simulink model "attitude_sysid"  (R2018a)
settings: Solver=VariableStepAuto  StartTime=0.0  StopTime=40  RelTol=1e-3
undefined symbols (not defined in the file): drone, simulation_sampling_ts
libraries: simulink x4
settings Model: Creator=ros  LastModifiedBy=ros

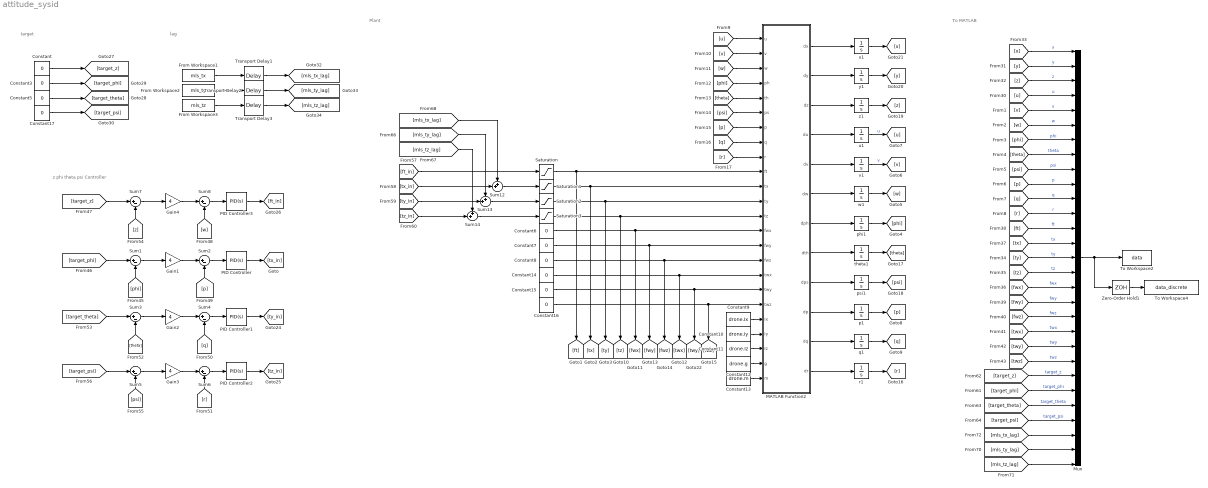
== system attitude_sysid ==
  note: Plant
  note: target
  note: lag
  note: z phi theta psi Controller
  note: To MATLAB
  Constant{,3,5..8,14..17} (10 alike) : Constant  Value=0
  Constant10 : Constant  Value=drone.Iy
  Constant11 : Constant  Value=drone.Iz
  Constant12 : Constant  Value=drone.g
  Constant13 : Constant  Value=drone.m
  Constant9 : Constant  Value=drone.Ix
  From Workspace1 : FromWorkspace  VariableName=mls_tx  SampleTime=0
  From Workspace2 : FromWorkspace  VariableName=mls_ty  SampleTime=0
  From Workspace3 : FromWorkspace  VariableName=mls_tz  SampleTime=0
  Gain{1..4} (4 alike) : Gain  Gain=4
  MATLAB Function2 : MATLAB Function  TreatAsAtomicUnit=on
  Mux : Mux  Inputs=29
  PID Controller : simulink/Continuous/PID Controller  Controller=PID  TimeDomain=Continuous-time  SampleTime=-1  IntegratorMethod=Forward Euler  FilterMethod=Forward Euler  Form=Parallel  UseFilter=on  ControllerParametersSource=internal  P=1.5  I=1.5  D=0  N=100  InitialConditionSource=internal  InitialConditionForIntegrator=0  InitialConditionForFilter=0  ExternalReset=none  LimitOutput=off  UpperSaturationLimit=inf  LowerSaturationLimit=-inf  LinearizeAsGain=on  AntiWindupMode=none  Kb=1  TrackingMode=off  Kt=1  PParamMin=[]  PParamMax=[]  IParamMin=[]  IParamMax=[]  DParamMin=[]  DParamMax=[]  NParamMin=[]  NParamMax=[]  KbParamMin=[]  KbParamMax=[]  KtParamMin=[]  KtParamMax=[]  POutMin=[]  POutMax=[]  IOutMin=[]  IOutMax=[]  DOutMin=[]  DOutMax=[]  NOutMin=[]  NOutMax=[]  KbOutMin=[]  KbOutMax=[]  KtOutMin=[]  KtOutMax=[]  IntegratorOutMin=[]  IntegratorOutMax=[]  FilterOutMin=[]  FilterOutMax=[]  SumOutMin=[]  SumOutMax=[]  SumI1OutMin=[]  SumI1OutMax=[]  SumI2OutMin=[]  SumI2OutMax=[]  SumI3OutMin=[]  SumI3OutMax=[]  SumDOutMin=[]  SumDOutMax=[]  SaturationOutMin=[]  SaturationOutMax=[]  IntegratorContinuousStateAttributes=''  IntegratorStateMustResolveToSignalObject=off  IntegratorRTWStateStorageClass=Auto  FilterContinuousStateAttributes=''  FilterStateMustResolveToSignalObject=off  FilterRTWStateStorageClass=Auto  DifferentiatorICPrevScaledInput=0  DifferentiatorOutMin=[]  DifferentiatorOutMax=[]  FilterDiffOutCoefMin=[]  FilterDiffOutCoefMax=[]  SumDenOutMin=[]  SumDenOutMax=[]  SumNumOutMin=[]  SumNumOutMax=[]  ReciprocalOutMin=[]  ReciprocalOutMax=[]  DivideOutMin=[]  DivideOutMax=[]  TunerSelectOption=Transfer Function Based (PID Tuner App)
  PID Controller1 : simulink/Continuous/PID Controller  Controller=PID  TimeDomain=Continuous-time  SampleTime=-1  IntegratorMethod=Forward Euler  FilterMethod=Forward Euler  Form=Parallel  UseFilter=on  ControllerParametersSource=internal  P=1.5  I=1.5  D=0  N=100  InitialConditionSource=internal  InitialConditionForIntegrator=0  InitialConditionForFilter=0  ExternalReset=none  LimitOutput=off  UpperSaturationLimit=inf  LowerSaturationLimit=-inf  LinearizeAsGain=on  AntiWindupMode=none  Kb=1  TrackingMode=off  Kt=1  PParamMin=[]  PParamMax=[]  IParamMin=[]  IParamMax=[]  DParamMin=[]  DParamMax=[]  NParamMin=[]  NParamMax=[]  KbParamMin=[]  KbParamMax=[]  KtParamMin=[]  KtParamMax=[]  POutMin=[]  POutMax=[]  IOutMin=[]  IOutMax=[]  DOutMin=[]  DOutMax=[]  NOutMin=[]  NOutMax=[]  KbOutMin=[]  KbOutMax=[]  KtOutMin=[]  KtOutMax=[]  IntegratorOutMin=[]  IntegratorOutMax=[]  FilterOutMin=[]  FilterOutMax=[]  SumOutMin=[]  SumOutMax=[]  SumI1OutMin=[]  SumI1OutMax=[]  SumI2OutMin=[]  SumI2OutMax=[]  SumI3OutMin=[]  SumI3OutMax=[]  SumDOutMin=[]  SumDOutMax=[]  SaturationOutMin=[]  SaturationOutMax=[]  IntegratorContinuousStateAttributes=''  IntegratorStateMustResolveToSignalObject=off  IntegratorRTWStateStorageClass=Auto  FilterContinuousStateAttributes=''  FilterStateMustResolveToSignalObject=off  FilterRTWStateStorageClass=Auto  DifferentiatorICPrevScaledInput=0  DifferentiatorOutMin=[]  DifferentiatorOutMax=[]  FilterDiffOutCoefMin=[]  FilterDiffOutCoefMax=[]  SumDenOutMin=[]  SumDenOutMax=[]  SumNumOutMin=[]  SumNumOutMax=[]  ReciprocalOutMin=[]  ReciprocalOutMax=[]  DivideOutMin=[]  DivideOutMax=[]  TunerSelectOption=Transfer Function Based (PID Tuner App)
  PID Controller2 : simulink/Continuous/PID Controller  Controller=PID  TimeDomain=Continuous-time  SampleTime=-1  IntegratorMethod=Forward Euler  FilterMethod=Forward Euler  Form=Parallel  UseFilter=on  ControllerParametersSource=internal  P=1.5  I=1.5  D=0  N=100  InitialConditionSource=internal  InitialConditionForIntegrator=0  InitialConditionForFilter=0  ExternalReset=none  LimitOutput=off  UpperSaturationLimit=inf  LowerSaturationLimit=-inf  LinearizeAsGain=on  AntiWindupMode=none  Kb=1  TrackingMode=off  Kt=1  PParamMin=[]  PParamMax=[]  IParamMin=[]  IParamMax=[]  DParamMin=[]  DParamMax=[]  NParamMin=[]  NParamMax=[]  KbParamMin=[]  KbParamMax=[]  KtParamMin=[]  KtParamMax=[]  POutMin=[]  POutMax=[]  IOutMin=[]  IOutMax=[]  DOutMin=[]  DOutMax=[]  NOutMin=[]  NOutMax=[]  KbOutMin=[]  KbOutMax=[]  KtOutMin=[]  KtOutMax=[]  IntegratorOutMin=[]  IntegratorOutMax=[]  FilterOutMin=[]  FilterOutMax=[]  SumOutMin=[]  SumOutMax=[]  SumI1OutMin=[]  SumI1OutMax=[]  SumI2OutMin=[]  SumI2OutMax=[]  SumI3OutMin=[]  SumI3OutMax=[]  SumDOutMin=[]  SumDOutMax=[]  SaturationOutMin=[]  SaturationOutMax=[]  IntegratorContinuousStateAttributes=''  IntegratorStateMustResolveToSignalObject=off  IntegratorRTWStateStorageClass=Auto  FilterContinuousStateAttributes=''  FilterStateMustResolveToSignalObject=off  FilterRTWStateStorageClass=Auto  DifferentiatorICPrevScaledInput=0  DifferentiatorOutMin=[]  DifferentiatorOutMax=[]  FilterDiffOutCoefMin=[]  FilterDiffOutCoefMax=[]  SumDenOutMin=[]  SumDenOutMax=[]  SumNumOutMin=[]  SumNumOutMax=[]  ReciprocalOutMin=[]  ReciprocalOutMax=[]  DivideOutMin=[]  DivideOutMax=[]  TunerSelectOption=Transfer Function Based (PID Tuner App)
  PID Controller3 : simulink/Continuous/PID Controller  Controller=PID  TimeDomain=Continuous-time  SampleTime=-1  IntegratorMethod=Forward Euler  FilterMethod=Forward Euler  Form=Parallel  UseFilter=on  ControllerParametersSource=internal  P=7  I=6  D=0.7  N=100  InitialConditionSource=internal  InitialConditionForIntegrator=0  InitialConditionForFilter=0  ExternalReset=none  LimitOutput=off  UpperSaturationLimit=inf  LowerSaturationLimit=-inf  LinearizeAsGain=on  AntiWindupMode=none  Kb=1  TrackingMode=off  Kt=1  PParamMin=[]  PParamMax=[]  IParamMin=[]  IParamMax=[]  DParamMin=[]  DParamMax=[]  NParamMin=[]  NParamMax=[]  KbParamMin=[]  KbParamMax=[]  KtParamMin=[]  KtParamMax=[]  POutMin=[]  POutMax=[]  IOutMin=[]  IOutMax=[]  DOutMin=[]  DOutMax=[]  NOutMin=[]  NOutMax=[]  KbOutMin=[]  KbOutMax=[]  KtOutMin=[]  KtOutMax=[]  IntegratorOutMin=[]  IntegratorOutMax=[]  FilterOutMin=[]  FilterOutMax=[]  SumOutMin=[]  SumOutMax=[]  SumI1OutMin=[]  SumI1OutMax=[]  SumI2OutMin=[]  SumI2OutMax=[]  SumI3OutMin=[]  SumI3OutMax=[]  SumDOutMin=[]  SumDOutMax=[]  SaturationOutMin=[]  SaturationOutMax=[]  IntegratorContinuousStateAttributes=''  IntegratorStateMustResolveToSignalObject=off  IntegratorRTWStateStorageClass=Auto  FilterContinuousStateAttributes=''  FilterStateMustResolveToSignalObject=off  FilterRTWStateStorageClass=Auto  DifferentiatorICPrevScaledInput=0  DifferentiatorOutMin=[]  DifferentiatorOutMax=[]  FilterDiffOutCoefMin=[]  FilterDiffOutCoefMax=[]  SumDenOutMin=[]  SumDenOutMax=[]  SumNumOutMin=[]  SumNumOutMax=[]  ReciprocalOutMin=[]  ReciprocalOutMax=[]  DivideOutMin=[]  DivideOutMax=[]  TunerSelectOption=Transfer Function Based (PID Tuner App)
  Saturation{,1..3} (4 alike) : Saturate  UpperLimit=30  LowerLimit=-100
  Sum{1..8} (8 alike) : Sum  Inputs=|+-
  Sum12 : Sum  Inputs=++|
  Sum13 : Sum  Inputs=++|
  Sum14 : Sum  Inputs=++|
  To Workspace2 : ToWorkspace  VariableName=data  SaveFormat=Timeseries  SampleTime=-1
  To Workspace4 : ToWorkspace  VariableName=data_discrete  SaveFormat=Timeseries  SampleTime=-1
  Transport Delay1 : TransportDelay  DelayTime=10
  Transport Delay2 : TransportDelay  DelayTime=10
  Transport Delay3 : TransportDelay  DelayTime=10
  Zero-Order Hold1 : ZeroOrderHold  SampleTime=simulation_sampling_ts
  p1 : Integrator
  phi1 : Integrator
  psi1 : Integrator
  q1 : Integrator
  r1 : Integrator
  theta1 : Integrator
  u1 : Integrator
  v1 : Integrator
  w1 : Integrator
  x1 : Integrator
  y1 : Integrator
  z1 : Integrator
  wires:
  [x] -> Mux/1  "x"
  [v] -> Mux/5  "v"
  [z] -> Mux/3  "z"
  [w] -> Mux/6  "w"
  [p] -> Mux/10  "p"
  [phi] -> Mux/7  "phi"
  [theta] -> Mux/8  "theta"
  [r] -> Mux/12  "r"
  [y] -> Mux/2  "y"
  [psi] -> Mux/9  "psi"
  [u] -> Mux/4  "u"
  [q] -> Mux/11  "q"
  Mux/1 -> Zero-Order Hold1/1, To Workspace2/1
  [ft] -> Mux/13  "ft"
  [tx] -> Mux/14  "tx"
  [ty] -> Mux/15  "ty"
  [tz] -> Mux/16  "tz"
  [fwx] -> Mux/17  "fwx"
  [fwy] -> Mux/18  "fwy"
  [fwz] -> Mux/19  "fwz"
  [twx] -> Mux/20  "twx"
  [twy] -> Mux/21  "twy"
  [twz] -> Mux/22  "twz"
  Zero-Order Hold1/1 -> To Workspace4/1
  [target_z] -> Mux/23  "target_z"
  [target_phi] -> Mux/24  "target_phi"
  [target_theta] -> Mux/25  "target_theta"
  [target_psi] -> Mux/26  "target_psi"
  [mls_tx_lag] -> Mux/27
  [mls_ty_lag] -> Mux/28
  [mls_tz_lag] -> Mux/29
  u1/1 -> [u]  "u"
  Saturation/1 -> [ft], MATLAB Function2/10(ft)
  phi1/1 -> [phi]
  y1/1 -> [y]
  [tz_in] -> Sum14/2
  Saturation3/1 -> [tz], MATLAB Function2/13(tz)
  v1/1 -> [v]  "v"
  [mls_tz_lag] -> Sum14/1
  MATLAB Function2/2(dy) -> y1/1
  [psi] -> MATLAB Function2/6(ps)
  Sum13/1 -> Saturation2/1
  Constant11/1 -> MATLAB Function2/22(Iz)
  Constant14/1 -> [twx], MATLAB Function2/17(twx)
  MATLAB Function2/6(dw) -> w1/1
  r1/1 -> [r]
  Constant9/1 -> MATLAB Function2/20(Ix)
  MATLAB Function2/9(dps) -> psi1/1
  [p] -> MATLAB Function2/7(p)
  Constant10/1 -> MATLAB Function2/21(Iy)
  psi1/1 -> [psi]
  Constant15/1 -> [twy], MATLAB Function2/18(twy)
  [mls_ty_lag] -> Sum13/1
  MATLAB Function2/8(dth) -> theta1/1
  [mls_tx_lag] -> Sum12/1
  [tx_in] -> Sum12/2
  x1/1 -> [x]
  MATLAB Function2/3(dz) -> z1/1
  Sum14/1 -> Saturation3/1
  MATLAB Function2/5(dv) -> v1/1
  [ty_in] -> Sum13/2
  MATLAB Function2/1(dx) -> x1/1
  z1/1 -> [z]
  MATLAB Function2/10(dp) -> p1/1
  q1/1 -> [q]
  Constant16/1 -> [twz], MATLAB Function2/19(twz)
  MATLAB Function2/11(dq) -> q1/1
  w1/1 -> [w]
  [theta] -> MATLAB Function2/5(th)
  Constant6/1 -> [fwx], MATLAB Function2/14(fwx)
  Constant12/1 -> MATLAB Function2/23(g)
  Saturation2/1 -> [ty], MATLAB Function2/12(ty)
  [q] -> MATLAB Function2/8(q)
  Constant8/1 -> [fwz], MATLAB Function2/16(fwz)
  theta1/1 -> [theta]
  Sum12/1 -> Saturation1/1
  MATLAB Function2/4(du) -> u1/1
  Saturation1/1 -> [tx], MATLAB Function2/11(tx)
  [u] -> MATLAB Function2/1(u)
  MATLAB Function2/12(dr) -> r1/1
  [phi] -> MATLAB Function2/4(ph)
  Constant7/1 -> [fwy], MATLAB Function2/15(fwy)
  MATLAB Function2/7(dph) -> phi1/1
  Constant13/1 -> MATLAB Function2/24(m)
  [r] -> MATLAB Function2/9(r)
  [ft_in] -> Saturation/1
  p1/1 -> [p]
  [w] -> MATLAB Function2/3(w)
  [v] -> MATLAB Function2/2(v)
  From Workspace2/1 -> Transport Delay2/1
  Transport Delay2/1 -> [mls_ty_lag]
  Constant5/1 -> [target_theta]
  Constant/1 -> [target_z]
  Transport Delay3/1 -> [mls_tz_lag]
  From Workspace3/1 -> Transport Delay3/1
  From Workspace1/1 -> Transport Delay1/1
  Constant3/1 -> [target_phi]
  Transport Delay1/1 -> [mls_tx_lag]
  Constant17/1 -> [target_psi]
  Gain4/1 -> Sum8/1
  Sum8/1 -> PID Controller3/1
  Sum5/1 -> Gain3/1
  Gain1/1 -> Sum2/1
  [q] -> Sum4/2
  Sum2/1 -> PID Controller/1
  PID Controller1/1 -> [ty_in]
  Sum1/1 -> Gain1/1
  [phi] -> Sum1/2
  [target_z] -> Sum7/1
  [psi] -> Sum5/2
  Sum7/1 -> Gain4/1
  [target_theta] -> Sum3/1
  [p] -> Sum2/2
  [w] -> Sum8/2
  Sum4/1 -> PID Controller1/1
  Sum6/1 -> PID Controller2/1
  Sum3/1 -> Gain2/1
  Gain3/1 -> Sum6/1
  [target_phi] -> Sum1/1
  [r] -> Sum6/2
  PID Controller3/1 -> [ft_in]
  [z] -> Sum7/2
  PID Controller2/1 -> [tz_in]
  [theta] -> Sum3/2
  PID Controller/1 -> [tx_in]
  [target_psi] -> Sum5/1
  Gain2/1 -> Sum4/1

== matlab function attitude_sysid/MATLAB Function2 ==
  data: u input; v input; dx output; w input; ph input; th input; ps input; p input; q input; r input; ft input; tx input; ty input; tz input; fwx input; fwy input; fwz input; twx input; twy input; twz input; dy output; dz output; du output; dv output; dw output; dph output; dth output; dps output; dp output; dq output; dr output; Ix input; Iy input; Iz input; g input; m input
function [dx, dy, dz, du, dv, dw, dph, dth, dps, dp, dq, dr] = fcn(u, v, w, ph, th, ps, p, q, r, ft, tx, ty, tz, fwx, fwy, fwz, twx, twy, twz, Ix, Iy, Iz, g, m)

dx = w*(sin(ph)*sin(ps) + cos(ph)*cos(ps)*sin(th)) - v*(cos(ph)*sin(ps) - cos(ps)*sin(ph)*sin(th)) + u*(cos(ps)*cos(th));
dy = v*(cos(ph)*cos(ps) + sin(ph)*sin(ps)*sin(th)) - w*(cos(ps)*sin(ph) - cos(ph)*sin(ps)*sin(th)) + u*(cos(th)*sin(ps));
dz = w*(cos(ph)*cos(th)) - u*(sin(th)) + v*(cos(th)*sin(ph));
du = r*v - q*w + g*(sin(th)) + fwx / m;
dv = p*w - r*u - g*(sin(ph)*cos(th)) + fwy / m;
dw = q*u - p*v - g*(cos(th)*cos(ph)) + (fwz + ft) / m;
dph = p + r*(cos(ph)*tan(th)) + q*(sin(ph)*tan(th));
dth = q*(cos(th)) - r*(sin(ph));
dps = r*(cos(ph)/cos(th)) + q*(sin(ph)/cos(th));
dp = r*q*(Iy - Iz)/Ix + (tx + twx)/Ix;
dq = p*r*(Iz - Ix)/Iy + (ty + twy)/Iy;
dr = p*q*(Ix - Iy)/Iz + (tz + twz)/Iz;
